simulink model "car_xxl"  (Simulink 6.1)
settings: Solver=ode45  StartTime=0.0  StopTime=50.0  RelTol=1e-3
libraries: simulink_extras x1, fuzblock x1
settings Model: LastModifiedBy=dyb
settings DataIOCC: SignalLoggingName=sigsOut
settings HardwareCC: TargetUnknown=on

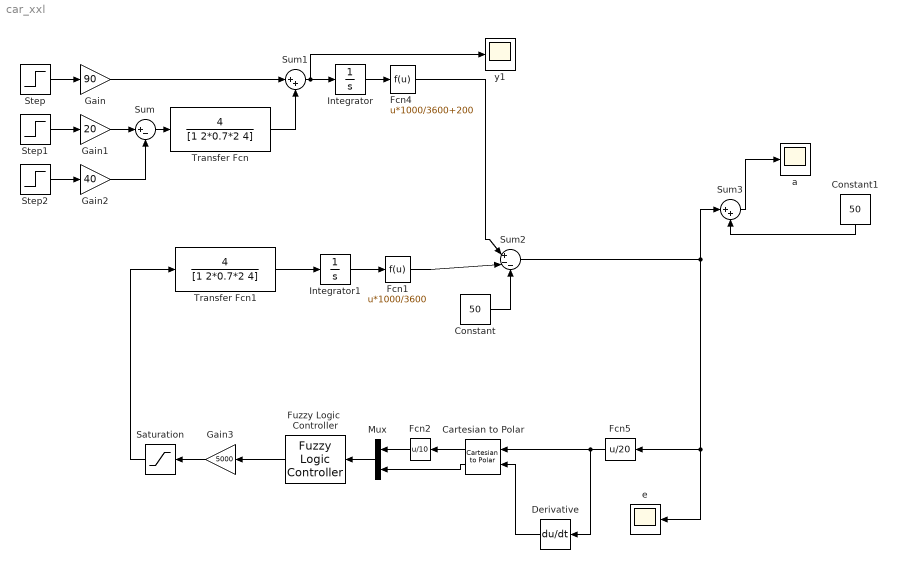
== system car_xxl ==
  Cartesian to Polar : simulink_extras/Transformations/Cartesian to Polar  Orientation=left
  Constant : Constant  Value=50
  Constant1 : Constant  Orientation=down  Value=50
  Derivative : Derivative  Orientation=left
  Fcn1 : Fcn  Expr=u*1000/3600
  Fcn2 : Fcn  Orientation=left  Expr=u/10
  Fcn4 : Fcn  Expr=u*1000/3600+200
  Fcn5 : Fcn  Orientation=left  Expr=u/20
  Fuzzy Logic  Controller : fuzblock/Fuzzy Logic  Controller  Orientation=left  fis=carf5
  Gain : Gain  Gain=90  SaturateOnIntegerOverflow=on
  Gain1 : Gain  Gain=20  SaturateOnIntegerOverflow=on
  Gain2 : Gain  Gain=40  SaturateOnIntegerOverflow=on
  Gain3 : Gain  Orientation=left  Gain=5000  SaturateOnIntegerOverflow=on
  Integrator : Integrator
  Integrator1 : Integrator
  Mux : Mux  Orientation=left  Inputs=2
  Saturation : Saturate  Orientation=left  UpperLimit=200  LowerLimit=0
  Step : Step  Time=0  SampleTime=0
  Step1 : Step  Time=25  SampleTime=0
  Step2 : Step  Time=35  SampleTime=0
  Sum : Sum  Inputs=|+-  SaturateOnIntegerOverflow=on
  Sum1 : Sum  Inputs=|++  SaturateOnIntegerOverflow=on
  Sum2 : Sum  Inputs=|+--  SaturateOnIntegerOverflow=on
  Sum3 : Sum  Inputs=|++  SaturateOnIntegerOverflow=on
  Transfer Fcn : TransferFcn  Numerator=[4]  Denominator=[1 2*0.7*2 4]
  Transfer Fcn1 : TransferFcn  Numerator=[4]  Denominator=[1 2*0.7*2 4]
  a : Scope
      settings: YMin=143.762  YMax=158.894
  e : Scope
      settings: TimeRange=50  YMin=-20  YMax=160  SaveName=ScopeData5
  y1 : Scope
      settings: SaveName=ScopeData2
  wires:
  Step/1 -> Gain/1
  Step1/1 -> Gain1/1
  Step2/1 -> Gain2/1
  Sum/1 -> Transfer Fcn/1
  Integrator/1 -> Fcn4/1
  Constant/1 -> Sum2/3
  Sum2/1 -> Fcn5/1, e/1, Sum3/1
  Constant1/1 -> Sum3/2
  Sum3/1 -> a/1
  Derivative/1 -> Cartesian to Polar/2
  Cartesian to Polar/2 -> Mux/2
  Mux/1 -> Fuzzy Logic  Controller/1
  Fcn1/1 -> Sum2/2
  Fcn4/1 -> Sum2/1
  Integrator1/1 -> Fcn1/1
  Fcn5/1 -> Derivative/1, Cartesian to Polar/1
  Transfer Fcn1/1 -> Integrator1/1
  Transfer Fcn/1 -> Sum1/2
  Sum1/1 -> y1/1, Integrator/1
  Gain/1 -> Sum1/1
  Gain1/1 -> Sum/1
  Gain2/1 -> Sum/2
  Cartesian to Polar/1 -> Fcn2/1
  Fcn2/1 -> Mux/1
  Fuzzy Logic  Controller/1 -> Gain3/1
  Gain3/1 -> Saturation/1
  Saturation/1 -> Transfer Fcn1/1
